simulink model "chap6_9sim"  (Simulink 5.0)
settings: Solver=ode45  StartTime=0.0  StopTime=20  RelTol=1e-3
libraries: simulink x1
settings Model: LastModifiedBy=Administrator

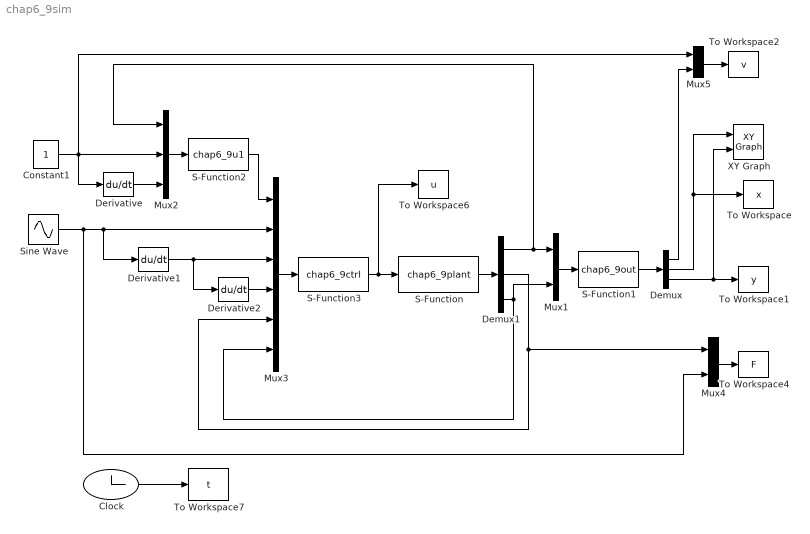
== system chap6_9sim ==
  Clock : Clock
      settings: Decimation=10
  Constant1 : Constant
  Demux : Demux  Outputs=3
  Demux1 : Demux  Outputs=3
  Derivative : Derivative
  Derivative1 : Derivative
  Derivative2 : Derivative
  Mux1 : Mux  Inputs=2
  Mux2 : Mux  Inputs=3
  Mux3 : Mux  Inputs=6
  Mux4 : Mux  Inputs=2
  Mux5 : Mux  Inputs=2
  S-Function : S-Function  FunctionName=chap6_9plant
  S-Function1 : S-Function  FunctionName=chap6_9out
  S-Function2 : S-Function  FunctionName=chap6_9u1
  S-Function3 : S-Function  FunctionName=chap6_9ctrl
  Sine Wave : Sin  SampleTime=0
  To Workspace : ToWorkspace  VariableName=x  SampleTime=-1  SaveFormat=Array
  To Workspace1 : ToWorkspace  VariableName=y  SampleTime=-1  SaveFormat=Array
  To Workspace2 : ToWorkspace  VariableName=v  SampleTime=-1  SaveFormat=Array
  To Workspace4 : ToWorkspace  VariableName=F  SampleTime=-1  SaveFormat=Array
  To Workspace6 : ToWorkspace  VariableName=u  SampleTime=-1  SaveFormat=Array
  To Workspace7 : ToWorkspace  VariableName=t  SampleTime=-1  SaveFormat=Array
  XY Graph : simulink/Sinks/XY Graph  xmin=0  xmax=20  ymin=-3  ymax=1.5  st=-1
  wires:
  S-Function/1 -> Demux1/1
  Demux1/1 -> Mux1/1, Mux2/1
  Demux1/3 -> Mux3/6, Mux1/2
  S-Function1/1 -> Demux/1
  Constant1/1 -> Derivative/1, Mux2/2, Mux5/1
  Derivative/1 -> Mux2/3
  Mux2/1 -> S-Function2/1
  Demux1/2 -> Mux4/1, Mux3/5
  S-Function3/1 -> S-Function/1, To Workspace6/1
  S-Function2/1 -> Mux3/1
  Sine Wave/1 -> Mux3/2, Derivative1/1, Mux4/2
  Derivative1/1 -> Mux3/3, Derivative2/1
  Derivative2/1 -> Mux3/4
  Mux3/1 -> S-Function3/1
  Mux1/1 -> S-Function1/1
  Clock/1 -> To Workspace7/1
  Mux4/1 -> To Workspace4/1
  Demux/3 -> To Workspace1/1, XY Graph/2
  Demux/2 -> To Workspace/1, XY Graph/1
  Demux/1 -> Mux5/2
  Mux5/1 -> To Workspace2/1
